simulink model "EnvT_VD"  (R2016b)
settings: configuration reference "CodeGenConfigSet" (kept outside this file)
values from neighbouring files (symbols this model uses):
  EnvT_facPT1_C = Calibration.Parameter    [init_EnvT_VD.m]
  EnvT_RmpSlpNeg_C = Calibration.Parameter    [init_EnvT_VD.m]
  EnvT_RmpSlpPos_C = Calibration.Parameter    [init_EnvT_VD.m]
  EnvT_tTransStgDfl_C = Calibration.Parameter    [init_EnvT_VD.m]
  SigTst_swtEnvT_C = Calibration.Parameter    [init_EnvT_VD.m]
  SigTst_tEnvT_C = Calibration.Parameter    [init_EnvT_VD.m]
undefined symbols (not defined in the file or in its folder): CEngDst_switch_conv, EnvT_VD_DT, Switch_conv
libraries: CXLib x4
settings Model: Creator=lenovo  LastModifiedBy=lenovo
settings ConfigSetRef: SourceLocation=Base Workspace

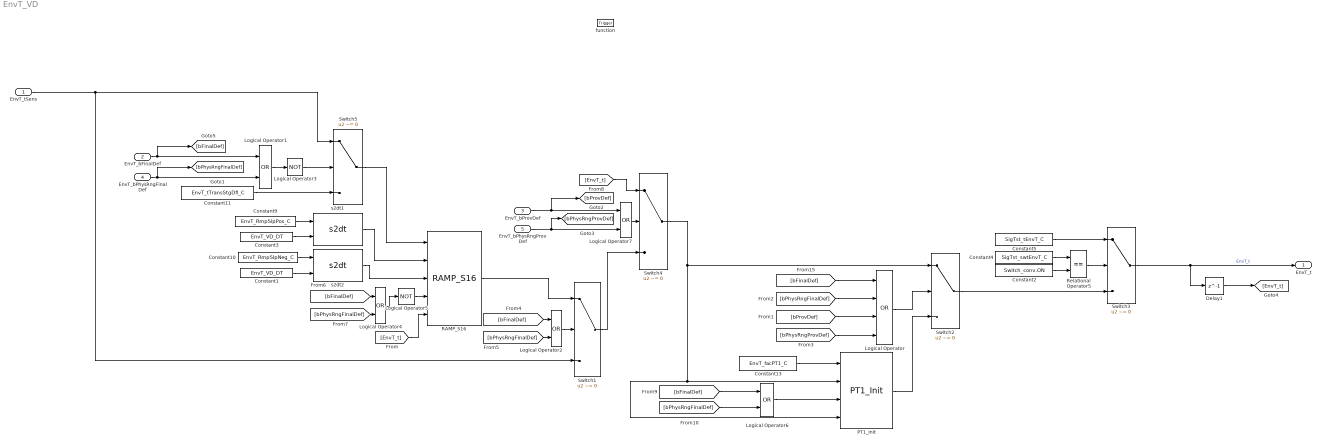
== system EnvT_VD ==
  EnvT_tSens : Inport  Tag=deg  Description=Raw physical value  OutMin=-200  OutMax=200  OutDataTypeStr=Temp_deg
  EnvT_bFinalDef : Inport  Description=Environment temperature sensor finally defect flag  Port=2  OutMin=0  OutMax=1  OutDataTypeStr=boolean
  EnvT_bProvDef : Inport  Description=Environment temperature sensor temporary defect flag  Port=3  OutMin=0  OutMax=1  OutDataTypeStr=boolean
  EnvT_bPhysRngFinalDef : Inport  Description=Environment temperature sensor physical range finally defect  Port=4  OutMin=0  OutMax=1  OutDataTypeStr=boolean
  EnvT_bPhysRngProvDef : Inport  Description=Environment temperature sensor physical range temporary defect  Port=5  OutMin=0  OutMax=1  OutDataTypeStr=boolean
  function : TriggerPort  TriggerType=function-call  VariantControl=Variant
  Constant1 : Constant  Value=EnvT_VD_DT  OutDataTypeStr=Debounce_ms
  Constant10 : Constant  RequirementInfo={'other' 'CEngDsT_requirements.doc' '@Simulink_requirement_item_8' 'true' '冷却水温故障时斜坡至默认值' '' } %GIDa_3c79a588_fddf_46b2_ba19_7c633d252bc7  Value=EnvT_RmpSlpNeg_C  SampleTime=-1
  Constant11 : Constant  RequirementInfo={'other' 'CEngDsT_requirements.doc' '@Simulink_requirement_item_8' 'true' '冷却水温故障时斜坡至默认值' '' } %GIDa_351ec4bd_c5c4_4df6_9e3d_5bce2027ce9c  Value=EnvT_tTransStgDfl_C  SampleTime=-1
  Constant13 : Constant  Value=EnvT_facPT1_C  SampleTime=-1
  Constant2 : Constant  RequirementInfo={'other' 'APP_requirements.doc' '@Simulink_requirement_item_25' 'true' '手动开关' '' } %GIDa_a4c6fbfa_e4d0_4cfd_a2d7_07ef0d1cd442  Value=Switch_conv.ON  OutDataTypeStr=Inherit: Inherit via back propagation
  Constant3 : Constant  Value=EnvT_VD_DT  OutDataTypeStr=Debounce_ms
  Constant4 : Constant  RequirementInfo={'other' 'CEngDsT_requirements.doc' '@Simulink_requirement_item_6' 'true' '手动冷却水温值' '' } %GIDa_4e0e5620_854f_4a76_b214_9603c2ca722d  Value=SigTst_swtEnvT_C  SampleTime=-1
  Constant5 : Constant  RequirementInfo={'other' 'CEngDsT_requirements.doc' '@Simulink_requirement_item_6' 'true' '手动冷却水温值' '' } %GIDa_82cb50da_511d_4bf8_8c94_666c08f797e1  Value=SigTst_tEnvT_C  SampleTime=-1
  Constant9 : Constant  RequirementInfo={'other' 'CEngDsT_requirements.doc' '@Simulink_requirement_item_8' 'true' '冷却水温故障时斜坡至默认值' '' } %GIDa_28d8354b_8987_4c0d_82a8_5b55700b0092  Value=EnvT_RmpSlpPos_C  SampleTime=-1
  Delay1 : Delay  DialogController=Simulink.DDGSource  DelayLength=1  InitialCondition=0
  Logical Operator : Logic  Operator=OR  Inputs=4  OutDataTypeStr=boolean
  Logical Operator{1..2,4,6..7} (5 alike) : Logic  Operator=OR  OutDataTypeStr=boolean
  Logical Operator3 : Logic  Operator=NOT  AllPortsSameDT=off  OutDataTypeStr=boolean
  Logical Operator5 : Logic  Operator=NOT  AllPortsSameDT=off  OutDataTypeStr=boolean
  PT1_Init : CXLib/PT1_Init  offset=2731.4
  RAMP_S16 : CXLib/RAMP_S16  RequirementInfo={'other' 'CEngDsT_requirements.doc' '@Simulink_requirement_item_8' 'true' '冷却水温故障时斜坡至默认值' '' } %GIDa_a3475fa9_f5b4_40fc_ba30_2f762bf5c985
  Relational Operator5 : RelationalOperator  Operator===  OutDataTypeStr=boolean  RndMeth=Simplest  InputSameDT=on
  Switch1 : Switch  Criteria=u2 ~= 0  InputSameDT=on
  Switch2 : Switch  RequirementInfo={'other' 'CEngDsT_requirements.doc' '@Simulink_requirement_item_5' 'true' '冷却水温滤波去抖动' '' } %GIDa_7d7598c4_9bac_4255_b4b9_195a7087391c  Criteria=u2 ~= 0  InputSameDT=on
  Switch3 : Switch  RequirementInfo={'other' 'CEngDsT_requirements.doc' '@Simulink_requirement_item_6' 'true' '手动冷却水温值' '' } %GIDa_d177f630_7cb1_4a9e_bfc8_0a220ac7779f  Criteria=u2 ~= 0  Threshold=CEngDst_switch_conv.OFF  InputSameDT=on
  Switch4 : Switch  Criteria=u2 ~= 0  InputSameDT=on
  Switch5 : Switch  Criteria=u2 ~= 0  InputSameDT=on
  s2dt1 : CXLib/s2dt
  s2dt2 : CXLib/s2dt
  EnvT_t : Outport  Tag=deg  Description=Environmental temperature  OutMin=-200  OutMax=200  OutDataTypeStr=Temp_deg
  wires:
  [EnvT_t] -> Switch4/1
  s2dt2/1 -> RAMP_S16/3
  Constant1/1 -> s2dt2/2
  Constant10/1 -> s2dt2/1
  s2dt1/1 -> RAMP_S16/2
  Constant3/1 -> s2dt1/2
  Constant9/1 -> s2dt1/1
  [EnvT_t] -> RAMP_S16/5
  Delay1/1 -> [EnvT_t]
  Logical Operator6/1 -> PT1_Init/3
  [bPhysRngFinalDef] -> Logical Operator6/2
  [bFinalDef] -> Logical Operator6/1
  Logical Operator5/1 -> RAMP_S16/4
  [bPhysRngFinalDef] -> Logical Operator4/2
  [bFinalDef] -> Logical Operator4/1
  [bPhysRngFinalDef] -> Logical Operator2/2
  [bFinalDef] -> Logical Operator2/1
  Constant2/1 -> Relational Operator5/2
  Constant4/1 -> Relational Operator5/1
  Relational Operator5/1 -> Switch3/2
  [bPhysRngProvDef] -> Logical Operator/4
  [bProvDef] -> Logical Operator/3
  [bPhysRngFinalDef] -> Logical Operator/2
  [bFinalDef] -> Logical Operator/1
  EnvT_bPhysRngProvDef/1 -> Logical Operator7/2, [bPhysRngProvDef]
  EnvT_bProvDef/1 -> Logical Operator7/1, [bProvDef]
  EnvT_bFinalDef/1 -> Logical Operator1/1, [bFinalDef]
  EnvT_bPhysRngFinalDef/1 -> Logical Operator1/2, [bPhysRngFinalDef]
  PT1_Init/1 -> Switch2/3
  RAMP_S16/1 -> Switch1/1
  Switch5/1 -> RAMP_S16/1
  Constant13/1 -> PT1_Init/1
  Constant5/1 -> Switch3/1
  Logical Operator4/1 -> Logical Operator5/1
  Logical Operator2/1 -> Switch1/2
  Logical Operator7/1 -> Switch4/2
  Logical Operator3/1 -> Switch5/2
  Logical Operator1/1 -> Logical Operator3/1
  Constant11/1 -> Switch5/3
  Switch3/1 -> EnvT_t/1, Delay1/1  "EnvT_t"
  Switch2/1 -> Switch3/3
  Logical Operator/1 -> Switch2/2
  Switch1/1 -> Switch4/3
  Switch4/1 -> Switch2/1, PT1_Init/4, PT1_Init/2
  EnvT_tSens/1 -> Switch5/1, Switch1/3
